simulink model "psbneutral"  (Simulink 6.0)
settings: Solver=VariableStepDiscrete  SolverMode=SingleTasking  StartTime=0.0  StopTime=10.0  MaxStep=1e-03  RelTol=1e-3  AbsTol=1e-6
libraries: powerlib2 x13
settings Model: Creator=patrice  LastModifiedBy=batserve  ExtModeTrigMode=oneshot  ExtModeArmWhenConnect=off  ExtModeAutoUpdateStatusClock=off
settings DataIOCC: LimitDataPoints=off  SignalLoggingName=sigsOut
settings OptimizationCC: BooleanDataType=off
settings DebuggingCC: SolverPrmCheckMsg=none
settings HardwareCC: TargetUnknown=on
settings RTWCC: TemplateMakefile=grt_unix.tmf

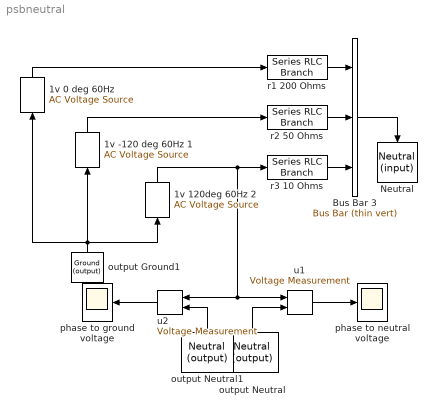
== system psbneutral ==
  1v -120 deg 60Hz 1 : powerlib2/Electrical Sources/AC Voltage Source  Tag=PoWeRsYsTeMbLoCk  Orientation=up  A=1  P=-120  F=60  stime=0  mesure=None  PSBOutputType=1
  "1v 0 deg 60Hz " : powerlib2/Electrical Sources/AC Voltage Source  Tag=PoWeRsYsTeMbLoCk  Orientation=up  A=1  P=0  F=60  stime=0  mesure=None  PSBOutputType=1
  1v 120deg 60Hz 2 : powerlib2/Electrical Sources/AC Voltage Source  Tag=PoWeRsYsTeMbLoCk  Orientation=up  A=1  P=120  F=60  stime=0  mesure=None  PSBOutputType=1
  Bus Bar 3 : powerlib2/Connectors/Bus Bar (thin vert)  Tag=PoWeRsYsTeMbLoCk  input=3  output=1  PSBOutputType=111111111111111111111111111111111111111111111111111111111111111111111111111111111111
  Neutral : powerlib2/Connectors/Neutral (input)  Tag=PoWeRsYsTeMbLoCk  Orientation=down  no=50
  output Ground1 : powerlib2/Connectors/Ground (output)  Tag=PoWeRsYsTeMbLoCk  Orientation=up  PSBOutputType=1
  output Neutral : powerlib2/Connectors/Neutral (output)  Tag=PoWeRsYsTeMbLoCk  Orientation=up  no=50  PSBOutputType=1
  output Neutral1 : powerlib2/Connectors/Neutral (output)  Tag=PoWeRsYsTeMbLoCk  Orientation=up  no=0  PSBOutputType=1
  phase to ground voltage : Scope
      settings: TickLabels=on  TimeRange=0.1  YMin=-1.2  YMax=1.2  DataFormat=Array
  phase to neutral voltage : Scope
      settings: TickLabels=on  TimeRange=0.1  YMin=-1.2  YMax=1.2  DataFormat=Array
  r1 200 Ohms : powerlib2/Elements/Series RLC Branch  Tag=PoWeRsYsTeMbLoCk  a=200  b=0  c=inf  mesure=None  PSBOutputType=1
  r2 50 Ohms : powerlib2/Elements/Series RLC Branch  Tag=PoWeRsYsTeMbLoCk  a=50  b=0  c=inf  mesure=None  PSBOutputType=1
  r3 10 Ohms : powerlib2/Elements/Series RLC Branch  Tag=PoWeRsYsTeMbLoCk  a=10  b=0  c=inf  mesure=None  PSBOutputType=1
  u1 : powerlib2/Measurements/Voltage Measurement  Tag=PoWeRsYsTeMmEaSuReMeNt  PhasorSimulation=off  OutputType=Magnitude  PSBOutputType=0  PSBequivalent=0
  u2 : powerlib2/Measurements/Voltage Measurement  Tag=PoWeRsYsTeMmEaSuReMeNt  Orientation=left  PhasorSimulation=off  OutputType=Magnitude  PSBOutputType=0  PSBequivalent=0
  wires:
  output Ground1/1 -> 1v -120 deg 60Hz 1/1, 1v 120deg 60Hz 2/1, "1v 0 deg 60Hz "/1
  "1v 0 deg 60Hz "/1 -> r1 200 Ohms/1
  r2 50 Ohms/1 -> Bus Bar 3/2
  r1 200 Ohms/1 -> Bus Bar 3/1
  1v -120 deg 60Hz 1/1 -> r2 50 Ohms/1
  Bus Bar 3/1 -> Neutral/1
  r3 10 Ohms/1 -> Bus Bar 3/3
  output Neutral/1 -> u1/2
  u1/1 -> phase to neutral voltage/1
  u2/1 -> phase to ground voltage/1
  output Neutral1/1 -> u2/2
  1v 120deg 60Hz 2/1 -> r3 10 Ohms/1, u2/1, u1/1
